simulink model "Problem_5"  (R2020a)
settings: Solver=VariableStepAuto  StartTime=0.0  StopTime=5  RelTol=1e-3
model workspace (MAT data in the model file):
  table_number = Simulink.Parameter
  table_number.Value = [1 2 3 4 5]
  table_number.DataType = 'auto'
  table_number.Dimensions = [1 5]
  table_value = Simulink.Parameter
  table_value.Value = [0.5 40 12 100 0.0009]
  table_value.DataType = 'auto'
  table_value.Dimensions = [1 5]
libraries: powerlib x6
settings Model: Creator=Saqlain  LastModifiedBy=Saqlain

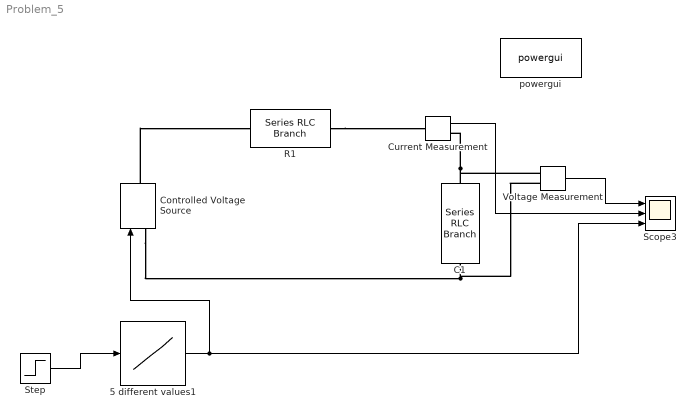
== system Problem_5 ==
  5 different values1 : Lookup_n-D  NumberOfTableDimensions=1  BreakpointsForDimension1=table_number  Table=table_value  InternalRulePriority=Speed  RndMeth=Simplest  InputSameDT=on
  C1 : powerlib/Elements/Series RLC Branch  LConnTagsString=__new0  RConnTagsString=__new0  BranchType=C  Resistance=10  Inductance=1e-3  SetiL0=off  InitialCurrent=0  Capacitance=0.01  Setx0=off  InitialVoltage=0  Measurements=None
  Controlled Voltage Source : powerlib/Electrical Sources/Controlled Voltage Source  Initialize=on  Source_Type=DC  Amplitude=0  Phase=0  Frequency=0  Measurements=None
  Current Measurement : powerlib/Measurements/Current Measurement  PhasorSimulation=off  OutputType=Complex  PSBequivalent=0
  R1 : powerlib/Elements/Series RLC Branch  LConnTagsString=__new0  RConnTagsString=__new0  BranchType=R  Resistance=10  Inductance=1e-3  SetiL0=off  InitialCurrent=0  Capacitance=1e-6  Setx0=off  InitialVoltage=0  Measurements=None
  Scope3 : Scope  NumInputPorts=3
  Step : Step  Time=2  SampleTime=0
  Voltage Measurement : powerlib/Measurements/Voltage Measurement  PhasorSimulation=off  OutputType=Complex  PSBequivalent=0
  powergui : powerlib/powergui  Priority=1  SimulationMode=Continuous  SampleTime=50e-6  frequency=60  Iterations=50  frequencyindice=0  Pbase=100e6  ErrMax=1e-4  UnitsV=kV  UnitsW=MW  buscounter=0  FunctionMessages=off  echomessages=off  EnableUseOfTLC=off  CurrentSourceSwitches=off  DisableSnubberDevices=off  DisableRonSwitches=off  DisableVfSwitches=off  DisplayEquations=off  AutomaticDiscreteSolvers=off  SolverType=Tustin/Backward Euler (TBE)  Interpol=off  ExternalGateDelay=off  methode=off  Ts=100  x0status=blocks  SPID=on  SwTol=0  HookPort=off  NonlinearTolerance=1e-4  nMaxIteration=100  ContinueOnMaxIteration=off  RestoreLinks=warning  ResistiveCurrentMeasurement=off  Frange=[0:2:500]  Ylog=off  Xlog=on  ShowGrid=off  save=off  variable=ZData  structure=0  ZoomFFT=off  StartTime=0.0  cycles=1  DisplayStyle=1  fundamental=60  FreqAxis=off  MaxFrequency=1000  frequencyindicesteady=1  RmsSteady=1  display=off
  wires:
  Voltage Measurement/1 -> Scope3/1
  Current Measurement/1 -> Scope3/2
  5 different values1/1 -> Scope3/3, Controlled Voltage Source/1
  Step/1 -> 5 different values1/1
  connections:
  Controlled Voltage Source/RConn1 -- R1/LConn1
  Controlled Voltage Source/LConn1 -- Voltage Measurement/LConn2 -- C1/RConn1
  R1/RConn1 -- Current Measurement/LConn1
  C1/LConn1 -- Current Measurement/RConn1 -- Voltage Measurement/LConn1
